simulink model "Normalisation11"  (R2018b)
settings: Solver=FixedStepDiscrete  StartTime=0.0  StopTime=10  RelTol=1e-3
undefined symbols (not defined in the file): gray
libraries: visionsources x1, dspmtrx3 x1
settings Model: Creator=Administrator  LastModifiedBy=Administrator
settings SolverCC: AutoInsertRateTranBlk=on
settings OptimizationCC: BlockReduction=off  ConditionallyExecuteInputs=off  DefaultParameterBehavior=Inlined
settings DebuggingCC: AlgebraicLoopMsg=error  SingleTaskRateTransMsg=error
settings HardwareCC: ProdBitPerPointer=32  ProdBitPerSizeT=32  ProdBitPerPtrDiffT=32  ProdLargestAtomicFloat=None  ProdIntDivRoundTo=Undefined  ProdEndianess=Unspecified  ProdWordSize=32  ProdHWDeviceType=ASIC/FPGA->ASIC/FPGA  TargetBitPerPointer=64  TargetBitPerSizeT=64  TargetBitPerPtrDiffT=64  TargetLongLongMode=on  TargetIntDivRoundTo=Zero  TargetEndianess=LittleEndian  TargetWordSize=64  TargetHWDeviceType=Custom Processor->MATLAB Host Computer  ProdEqTarget=off

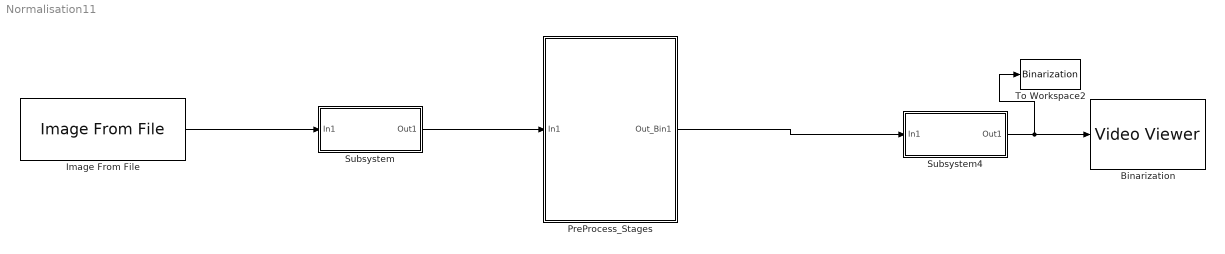
== system Normalisation11 ==
  Binarization : VideoViewer  colormapValue=gray(256)  FigPos=[203 867 376 593]
  Image From File : visionsources/Image From File  Tag=vipblks_nd  FileName=C:\Users\Administrator\Desktop\chapter\101_4.tif  imagePorts=One multidimensional signal  Ts=0.1  ImageDataType=uint8  Signed=on  WordLength=16  sdImageDataType=uint(8)  FractionLengthMode=User-defined  FractionLength=15  OutPortLabels=R|G|B
      settings: SourceProductName=Computer Vision System Toolbox
  PreProcess_Stages : Subsystem  TreatAsAtomicUnit=on
  Subsystem : Subsystem
  Subsystem4 : Subsystem
  To Workspace2 : ToWorkspace  VariableName=Binarization  SampleTime=-1
      settings: Save2DSignal=2-D array (concatenate along first dimension)
  wires:
  Image From File/1 -> Subsystem/1(In1)
  Subsystem/1(Out1) -> PreProcess_Stages/1(In1)
  Subsystem4/1(Out1) -> To Workspace2/1, Binarization/1
  PreProcess_Stages/1(Out_Bin1) -> Subsystem4/1(In1)

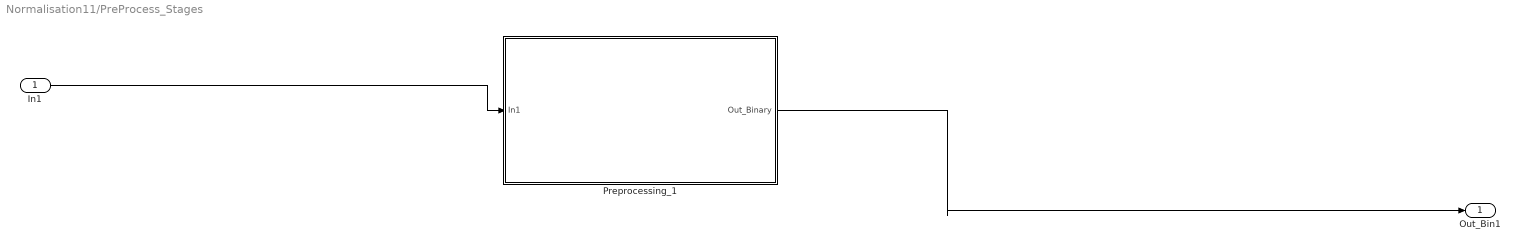
== system Normalisation11/PreProcess_Stages ==
  In1 : Inport
  Preprocessing_1 : Subsystem  TreatAsAtomicUnit=on
  Out_Bin1 : Outport
  wires:
  In1/1 -> Preprocessing_1/1(In1)
  Preprocessing_1/1(Out_Binary) -> Out_Bin1/1

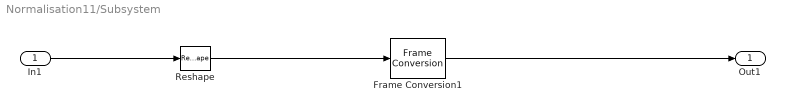
== system Normalisation11/Subsystem ==
  In1 : Inport
  Frame Conversion1 : FrameConversion  OutFrame=Sample-based
  Reshape : Reshape
  Out1 : Outport
  wires:
  Frame Conversion1/1 -> Out1/1
  Reshape/1 -> Frame Conversion1/1
  In1/1 -> Reshape/1

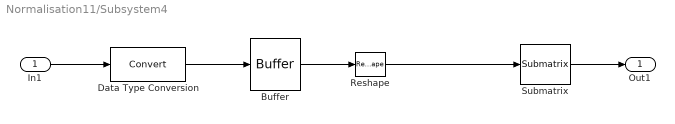
== system Normalisation11/Subsystem4 ==
  In1 : Inport
  Buffer : Buffer  N=8192  OutputFrames=off
  Data Type Conversion : DataTypeConversion
  Reshape : Reshape  OutputDimensionality=Customize  OutputDimensions=[128,64]
  Submatrix : dspmtrx3/Submatrix  RowSpan=Range of rows  RowStartMode=First  RowStartIndex=1  RowEndMode=Last  RowEndIndex=1  ColSpan=Range of columns  ColStartMode=First  ColStartIndex=1  ColEndMode=Last  ColEndIndex=1
  Out1 : Outport
  wires:
  Data Type Conversion/1 -> Buffer/1
  Buffer/1 -> Reshape/1
  Reshape/1 -> Submatrix/1
  Submatrix/1 -> Out1/1
  In1/1 -> Data Type Conversion/1

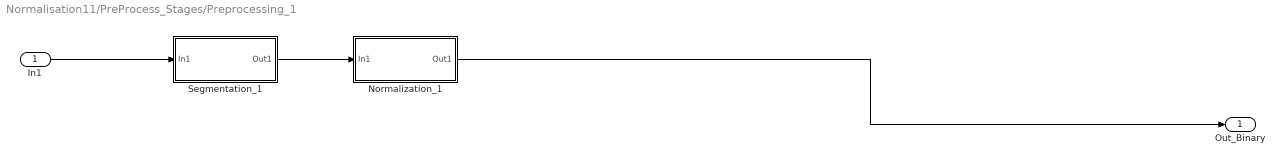
== system Normalisation11/PreProcess_Stages/Preprocessing_1 ==
  In1 : Inport
  Normalization_1 : Subsystem  TreatAsAtomicUnit=on
  Segmentation_1 : Subsystem  TreatAsAtomicUnit=on
  Out_Binary : Outport
  wires:
  Segmentation_1/1(Out1) -> Normalization_1/1(In1)
  In1/1 -> Segmentation_1/1(In1)
  Normalization_1/1(Out1) -> Out_Binary/1

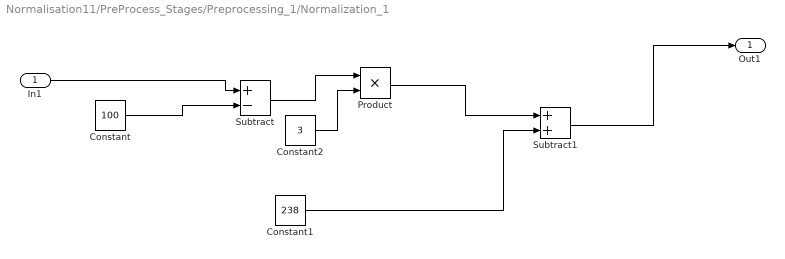
== system Normalisation11/PreProcess_Stages/Preprocessing_1/Normalization_1 ==
  In1 : Inport
  Constant : Constant  Value=100  OutDataTypeStr=uint8  SampleTime=-1
  Constant1 : Constant  Value=238  OutDataTypeStr=uint8  SampleTime=-1
  Constant2 : Constant  Value=3  OutDataTypeStr=uint8  SampleTime=-1
  Product : Product
  Subtract : Sum  Inputs=+-
  Subtract1 : Sum
  Out1 : Outport
  wires:
  In1/1 -> Subtract/1
  Product/1 -> Subtract1/1
  Constant1/1 -> Subtract1/2
  Subtract/1 -> Product/1
  Constant2/1 -> Product/2
  Subtract1/1 -> Out1/1
  Constant/1 -> Subtract/2

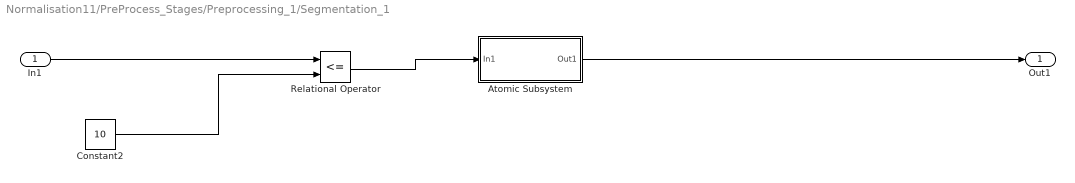
== system Normalisation11/PreProcess_Stages/Preprocessing_1/Segmentation_1 ==
  In1 : Inport
  Atomic Subsystem : Subsystem  TreatAsAtomicUnit=on
  Constant2 : Constant  Value=10  OutDataTypeStr=fixdt(1,16)  SampleTime=-1
  Relational Operator : RelationalOperator  Operator=<=  OutDataTypeStr=boolean  RndMeth=Nearest
  Out1 : Outport
  wires:
  Atomic Subsystem/1(Out1) -> Out1/1
  Relational Operator/1 -> Atomic Subsystem/1(In1)
  In1/1 -> Relational Operator/1
  Constant2/1 -> Relational Operator/2

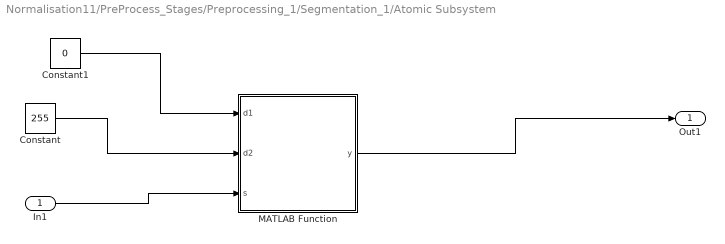
== system Normalisation11/PreProcess_Stages/Preprocessing_1/Segmentation_1/Atomic Subsystem ==
  In1 : Inport
  Constant : Constant  Value=255
  Constant1 : Constant  Value=0
  MATLAB Function : MATLAB Function  TreatAsAtomicUnit=on
  Out1 : Outport
  wires:
  In1/1 -> MATLAB Function/3(s)
  Constant1/1 -> MATLAB Function/1(d1)
  Constant/1 -> MATLAB Function/2(d2)
  MATLAB Function/1(y) -> Out1/1

== matlab function Normalisation11/PreProcess_Stages/Preprocessing_1/Segmentation_1/Atomic Subsystem/MATLAB Function ==
  data: d1 input; y output; d2 input; s input
function y = fcn(d1,d2,s)
%#codegen
if(s == true)
    y = uint8(d1);
else
    y = uint8(d2);
end
